simulink model "ES_simulation_models"  (R2022a)
settings: Solver=VariableStepAuto  StartTime=0.0  StopTime=4  RelTol=1e-3
values from neighbouring files (symbols this model uses):
  dt = 0.016    [ES_designing_control.m]
  KA = acker(MA_d_A,MA_d_B,[z1 z2])    [ES_designing_control.m]
  KA_I = acker(MA_d_A_I,MA_d_B_I,[z1 z2 z3])    [ES_designing_control.m]
  KB_I = acker(MB_d_A_I,MB_d_B_I,[z1 z2 z3])    [ES_designing_control.m]
  LA = acker(MA_d_A',MA_d_C',[z1_o z2_o])'    [ES_designing_control.m]
  LB = acker(MB_d_A',MB_d_C',[z1_o z2_o])'    [ES_designing_control.m]
  MA_A = [(-1*MA_b2/MA_b1) (-1*MA_b3/MA_b1);1 0]    [ES_designing_control.m]
  MA_B = [(MA_a1/MA_b1);0]    [ES_designing_control.m]
  MA_C = [0 1]    [ES_designing_control.m]
  MA_D = 0    [ES_designing_control.m]
  MA_d_A = MA_d_A_I(1:2,1:2)    [ES_designing_control.m]
  MA_d_B = MA_d_B_I(1:2)    [ES_designing_control.m]
  MA_d_C = MA_d_C_I(1:2)    [ES_designing_control.m]
  MB_A = [(-1*MB_b2/MB_b1) (-1*MB_b3/MB_b1);1 0]    [ES_designing_control.m]
  MB_B = [(MB_a1/MB_b1);0]    [ES_designing_control.m]
  MB_C = [0 1]    [ES_designing_control.m]
  MB_D = 0    [ES_designing_control.m]
  MB_d_A = MB_d_A_I(1:2,1:2)    [ES_designing_control.m]
  MB_d_B = MB_d_B_I(1:2)    [ES_designing_control.m]
  MB_d_C = MB_d_C_I(1:2)    [ES_designing_control.m]
undefined symbols (not defined in the file or in its folder): DiscIntNeverNeededParam
settings Model: Creator=DELL  LastModifiedBy=jvlsq
settings SolverCC: AlgebraicLoopSolver=TrustRegion
settings DebuggingCC: UnconnectedInputMsg=warning  UnconnectedOutputMsg=warning  UnconnectedLineMsg=warning  SFMachineParentedDataDiag=warning

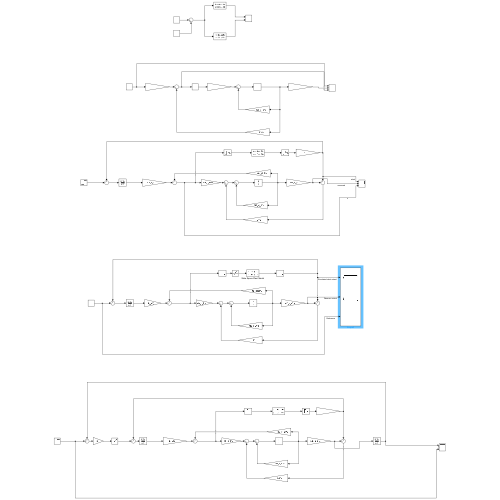
[thumbnail: Simulink's stored preview of the top-level diagram]
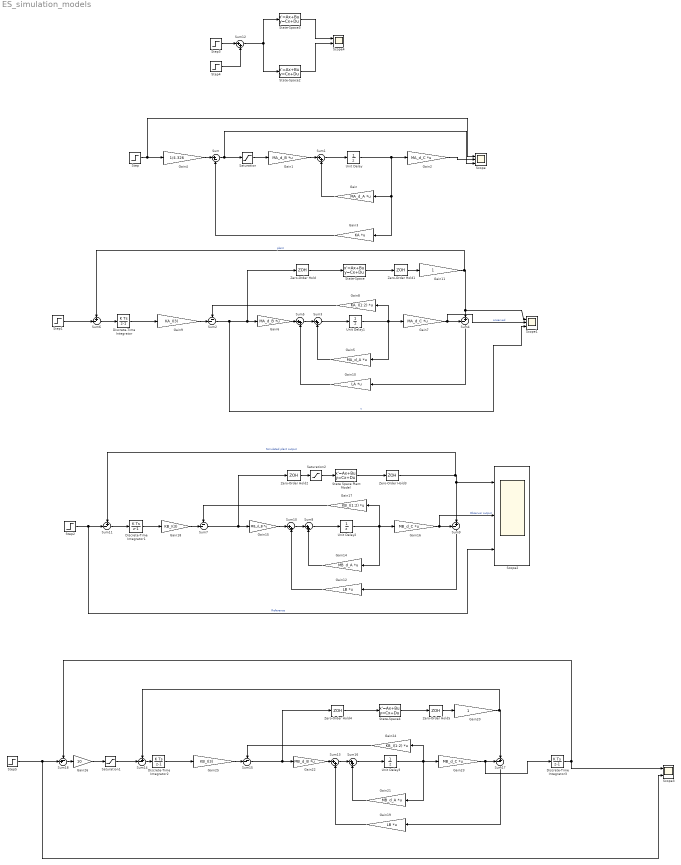
== system ES_simulation_models ==
  Discrete-Time Integrator{,1..3} (4 alike) : DiscreteIntegrator  SampleTime=dt  ICPrevOutput=DiscIntNeverNeededParam  ICPrevScaledInput=DiscIntNeverNeededParam
  Gain : Gain  Gain=MA_d_A  Multiplication=Matrix(K*u)
  Gain1 : Gain  Gain=MA_d_B  Multiplication=Matrix(K*u)
  Gain10 : Gain  Gain=LA  Multiplication=Matrix(K*u)
  Gain11 : Gain
  Gain12 : Gain  Gain=LB  Multiplication=Matrix(K*u)
  Gain14 : Gain  Gain=MB_d_A  Multiplication=Matrix(K*u)
  Gain15 : Gain  Gain=MB_d_B  Multiplication=Matrix(K*u)
  Gain16 : Gain  Gain=MB_d_C  Multiplication=Matrix(K*u)
  Gain17 : Gain  Gain=KB_I(1:2)  Multiplication=Matrix(K*u)
  Gain18 : Gain  Gain=KB_I(3)
  Gain19 : Gain  Gain=LB  Multiplication=Matrix(K*u)
  Gain2 : Gain  Gain=MA_d_C  Multiplication=Matrix(K*u)
  Gain20 : Gain
  Gain21 : Gain  Gain=MB_d_A  Multiplication=Matrix(K*u)
  Gain22 : Gain  Gain=MB_d_B  Multiplication=Matrix(K*u)
  Gain23 : Gain  Gain=MB_d_C  Multiplication=Matrix(K*u)
  Gain24 : Gain  Gain=KB_I(1:2)  Multiplication=Matrix(K*u)
  Gain25 : Gain  Gain=KB_I(3)
  Gain26 : Gain  Gain=10
  Gain3 : Gain  Gain=KA  Multiplication=Matrix(K*u)
  Gain4 : Gain  Gain=1/4.326
  Gain5 : Gain  Gain=MA_d_A  Multiplication=Matrix(K*u)
  Gain6 : Gain  Gain=MA_d_B  Multiplication=Matrix(K*u)
  Gain7 : Gain  Gain=MA_d_C  Multiplication=Matrix(K*u)
  Gain8 : Gain  Gain=KA_I(1:2)  Multiplication=Matrix(K*u)
  Gain9 : Gain  Gain=KA_I(3)
  Saturation : Saturate  UpperLimit=5  LowerLimit=-5
  Saturation1 : Saturate  UpperLimit=3  LowerLimit=-3
  Saturation2 : Saturate  UpperLimit=6  LowerLimit=-6
  Scope{,1..3} (4 alike) : Scope  NumInputPorts=3
  Scope4 : Scope  NumInputPorts=2
  State Space Plant Model : StateSpace  A=MB_A  B=MB_B  C=MB_C  D=MB_D  InitialCondition=0
  State-Space : StateSpace  A=MA_A  B=MA_B  C=MA_C  D=MA_D  InitialCondition=0
  State-Space2 : StateSpace  A=MA_A  B=MA_B  C=MA_C  D=MA_D  InitialCondition=0
  State-Space3 : StateSpace  A=MB_A  B=MB_B  C=MB_C  D=MB_D  InitialCondition=0
  State-Space4 : StateSpace  A=MB_A  B=MB_B  C=MB_C  D=MB_D  InitialCondition=0
  Step{,1..2,5} (4 alike) : Step  SampleTime=dt
  Step3 : Step  Time=2  After=4.5  SampleTime=dt
  Step4 : Step  Time=0  SampleTime=dt
  Sum : Sum  Inputs=|+-
  Sum{1,3,5,8,10,12..13,16} (8 alike) : Sum  Inputs=|++
  Sum11 : Sum  Inputs=+-|
  Sum14 : Sum  Inputs=+-|
  Sum15 : Sum  Inputs=--|
  Sum{4,9,17..18} (4 alike) : Sum  Inputs=-+|
  Sum2 : Sum  Inputs=--|
  Sum6 : Sum  Inputs=+-|
  Sum7 : Sum  Inputs=--|
  Unit Delay : UnitDelay  SampleTime=-1  HasFrameUpgradeWarning=on
  Unit Delay1 : UnitDelay  SampleTime=-1  HasFrameUpgradeWarning=on
  Unit Delay2 : UnitDelay  SampleTime=dt  HasFrameUpgradeWarning=on
  Unit Delay3 : UnitDelay  SampleTime=-1  HasFrameUpgradeWarning=on
  Zero-Order Hold{,1..5} (6 alike) : ZeroOrderHold  SampleTime=dt
  wires:
  Gain2/1 -> Scope/2
  Unit Delay/1 -> Gain3/1, Gain/1, Gain2/1
  Gain1/1 -> Sum1/1
  Sum1/1 -> Unit Delay/1
  Gain/1 -> Sum1/2
  Gain3/1 -> Sum/2
  Sum/1 -> Saturation/1, Scope/3
  Step/1 -> Gain4/1, Scope/1
  Gain4/1 -> Sum/1
  Saturation/1 -> Gain1/1
  Step1/1 -> Sum6/2
  Sum3/1 -> Unit Delay1/1
  Gain7/1 -> Scope1/2, Sum4/1  "onserved"
  Gain8/1 -> Sum2/1
  Unit Delay1/1 -> Gain5/1, Gain8/1, Gain7/1
  Gain5/1 -> Sum3/2
  Gain6/1 -> Sum5/1
  State-Space/1 -> Zero-Order Hold1/1
  Sum4/1 -> Gain10/1
  Zero-Order Hold1/1 -> Gain11/1
  Zero-Order Hold/1 -> State-Space/1
  Sum5/1 -> Sum3/1
  Gain10/1 -> Sum5/2
  Sum2/1 -> Scope1/3, Zero-Order Hold/1, Gain6/1  "u"
  Gain11/1 -> Sum6/1, Scope1/1, Sum4/2  "plant"
  Sum6/1 -> Discrete-Time Integrator/1
  Discrete-Time Integrator/1 -> Gain9/1
  Gain9/1 -> Sum2/2
  Zero-Order Hold2/1 -> Saturation2/1
  Sum10/1 -> Sum8/1
  Discrete-Time Integrator1/1 -> Gain18/1
  Sum7/1 -> Zero-Order Hold2/1, Gain15/1
  Gain14/1 -> Sum8/2
  Gain17/1 -> Sum7/1
  State Space Plant Model/1 -> Zero-Order Hold3/1
  Gain12/1 -> Sum10/2
  Sum9/1 -> Gain12/1
  Gain15/1 -> Sum10/1
  Step2/1 -> Scope2/3, Sum11/2  "Reference"
  Gain16/1 -> Scope2/2, Sum9/1  "Observer output"
  Sum8/1 -> Unit Delay2/1
  Unit Delay2/1 -> Gain14/1, Gain17/1, Gain16/1
  Gain18/1 -> Sum7/2
  Sum11/1 -> Discrete-Time Integrator1/1
  Zero-Order Hold3/1 -> Sum11/1, Sum9/2, Scope2/1  "Simulated plant output"
  State-Space2/1 -> Scope4/2
  Step4/1 -> Sum12/2
  Step3/1 -> Sum12/1
  Sum12/1 -> State-Space3/1, State-Space2/1
  State-Space3/1 -> Scope4/1
  Sum16/1 -> Unit Delay3/1
  Zero-Order Hold4/1 -> State-Space4/1
  Gain21/1 -> Sum16/2
  Unit Delay3/1 -> Gain21/1, Gain24/1, Gain23/1
  Sum15/1 -> Zero-Order Hold4/1, Gain22/1
  Sum13/1 -> Sum16/1
  Discrete-Time Integrator2/1 -> Gain25/1
  Gain20/1 -> Sum14/1, Sum17/2
  Sum14/1 -> Discrete-Time Integrator2/1
  Gain25/1 -> Sum15/2
  Gain23/1 -> Discrete-Time Integrator3/1, Sum17/1
  Step5/1 -> Sum18/2, Scope3/3
  Sum17/1 -> Gain19/1
  Gain24/1 -> Sum15/1
  State-Space4/1 -> Zero-Order Hold5/1
  Gain22/1 -> Sum13/1
  Zero-Order Hold5/1 -> Gain20/1
  Gain19/1 -> Sum13/2
  Sum18/1 -> Gain26/1
  Discrete-Time Integrator3/1 -> Sum18/1, Scope3/1
  Gain26/1 -> Saturation1/1
  Saturation1/1 -> Sum14/2
  Saturation2/1 -> State Space Plant Model/1
